simulink model "MovingAvg41"  (R2022a)
settings: Solver=FixedStepAuto  StartTime=0.0  StopTime=1500  FixedStep=1/3600  RelTol=1e-3
undefined symbols (not defined in the file or in its folder): sigbuilder_block
libraries: dspsrcs4 x1
settings Model: Creator=rupak  LastModifiedBy=rupak
settings ConfigComp: DVTestSuiteOptimization=Auto  DVDetectOutOfBounds=on  DVModelReferenceHarness=on  DVHarnessSource=Signal Editor

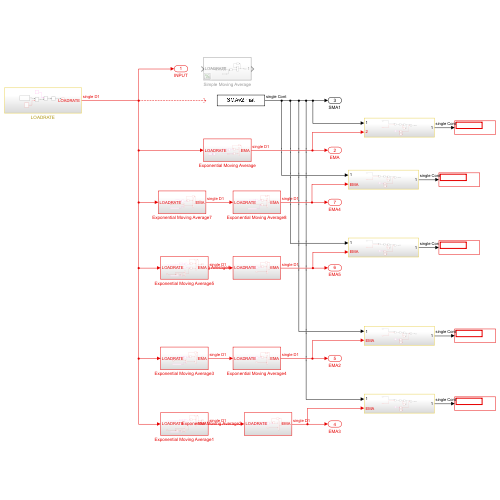
[thumbnail: Simulink's stored preview of the top-level diagram]
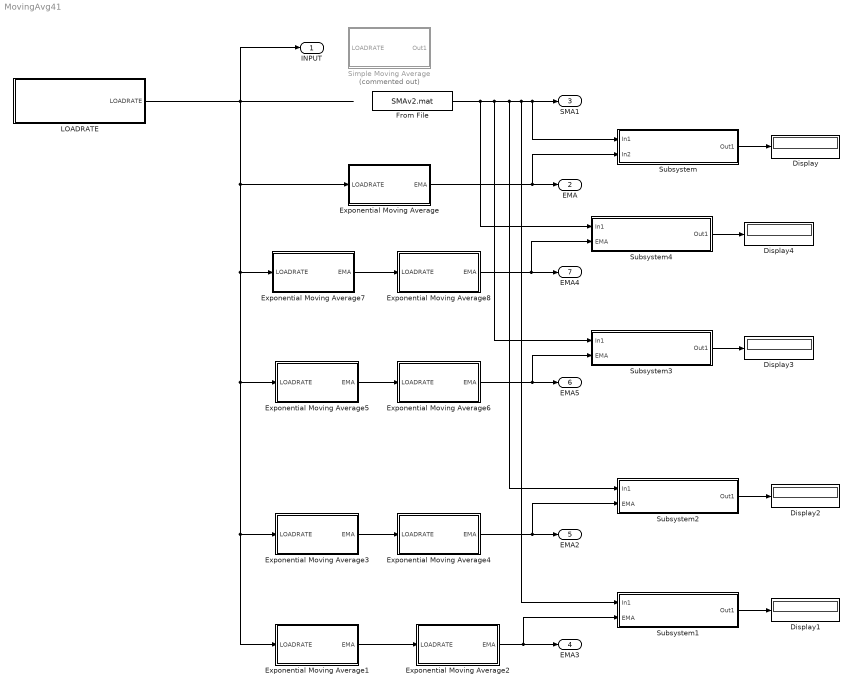
== system MovingAvg41 ==
  Display{,1..4} (5 alike) : Display
  Exponential Moving Average : Subsystem
  Exponential Moving Average1 : Subsystem
  Exponential Moving Average2 : Subsystem
  Exponential Moving Average3 : Subsystem
  Exponential Moving Average4 : Subsystem
  Exponential Moving Average5 : Subsystem
  Exponential Moving Average6 : Subsystem
  Exponential Moving Average7 : Subsystem
  Exponential Moving Average8 : Subsystem
  From File : FromFile  FileName=SMAv2.mat  SampleTime=0
  LOADRATE : Subsystem
  Simple Moving Average : Subsystem  Commented=on
  Subsystem : Subsystem
  Subsystem1 : Subsystem
  Subsystem2 : Subsystem
  Subsystem3 : Subsystem
  Subsystem4 : Subsystem
  INPUT : Outport
  EMA : Outport  Port=2
  SMA1 : Outport  Port=3
  EMA3 : Outport  Port=4
  EMA2 : Outport  Port=5
  EMA5 : Outport  Port=6
  EMA4 : Outport  Port=7
  wires:
  Exponential Moving Average/1(EMA) -> EMA/1, Subsystem/2(In2)
  Exponential Moving Average1/1(EMA) -> Exponential Moving Average2/1(LOADRATE)
  Exponential Moving Average2/1(EMA) -> EMA3/1, Subsystem1/2(EMA)
  LOADRATE/1(LOADRATE) -> INPUT/1, Exponential Moving Average3/1(LOADRATE), Exponential Moving Average1/1(LOADRATE), Exponential Moving Average5/1(LOADRATE), Exponential Moving Average7/1(LOADRATE), Exponential Moving Average/1(LOADRATE)
  Subsystem/1(Out1) -> Display/1
  Subsystem1/1(Out1) -> Display1/1
  Exponential Moving Average3/1(EMA) -> Exponential Moving Average4/1(LOADRATE)
  Exponential Moving Average4/1(EMA) -> Subsystem2/2(EMA), EMA2/1
  Subsystem2/1(Out1) -> Display2/1
  Exponential Moving Average8/1(EMA) -> Subsystem4/2(EMA), EMA4/1
  From File/1 -> Subsystem4/1(In1), Subsystem3/1(In1), Subsystem2/1(In1), Subsystem1/1(In1), Subsystem/1(In1), SMA1/1
  Subsystem4/1(Out1) -> Display4/1
  Exponential Moving Average5/1(EMA) -> Exponential Moving Average6/1(LOADRATE)
  Exponential Moving Average7/1(EMA) -> Exponential Moving Average8/1(LOADRATE)
  Exponential Moving Average6/1(EMA) -> EMA5/1, Subsystem3/2(EMA)
  Subsystem3/1(Out1) -> Display3/1

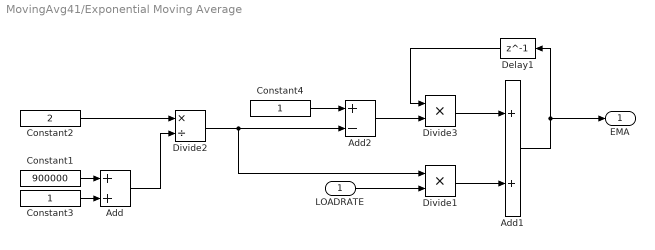
== system MovingAvg41/Exponential Moving Average ==
  LOADRATE : Inport
  Add : Sum
  Add1 : Sum
  Add2 : Sum  Inputs=+-
  Constant1 : Constant  Value=900000  OutDataTypeStr=single
  Constant2 : Constant  Value=2  OutDataTypeStr=single
  Constant3 : Constant  OutDataTypeStr=single
  Constant4 : Constant  OutDataTypeStr=single
  Delay1 : Delay  DelayLength=1  InitialCondition=60
  Divide1 : Product  Inputs=**
  Divide2 : Product  Inputs=*/
  Divide3 : Product  Inputs=**
  EMA : Outport
  wires:
  Add1/1 -> EMA/1, Delay1/1
  Divide1/1 -> Add1/2
  Constant2/1 -> Divide2/1
  Constant1/1 -> Add/1
  Constant3/1 -> Add/2
  Add/1 -> Divide2/2
  Delay1/1 -> Divide3/1
  Divide3/1 -> Add1/1
  Add2/1 -> Divide3/2
  Constant4/1 -> Add2/1
  Divide2/1 -> Add2/2, Divide1/1
  LOADRATE/1 -> Divide1/2

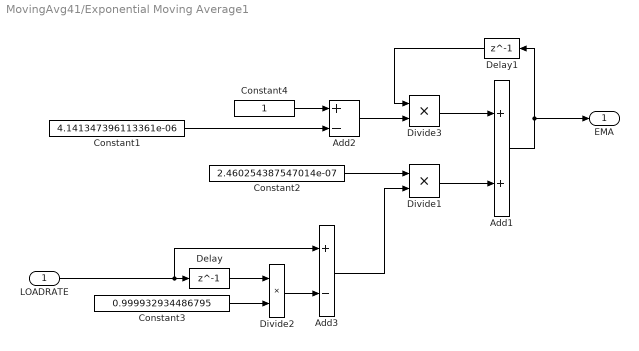
== system MovingAvg41/Exponential Moving Average1 ==
  LOADRATE : Inport
  Add1 : Sum
  Add2 : Sum  Inputs=+-
  Add3 : Sum  Inputs=+-
  Constant1 : Constant  Value=4.141347396113361e-06  OutDataTypeStr=single
  Constant2 : Constant  Value=2.460254387547014e-07  OutDataTypeStr=single
  Constant3 : Constant  Value=0.999932934486795  OutDataTypeStr=single
  Constant4 : Constant  OutDataTypeStr=single
  Delay : Delay  DelayLength=1  InitialCondition=60
  Delay1 : Delay  DelayLength=1  InitialCondition=0.000238234
  Divide1 : Product  Inputs=**
  Divide2 : Product  Inputs=**
  Divide3 : Product  Inputs=**
  EMA : Outport
  wires:
  Add1/1 -> EMA/1, Delay1/1
  Divide1/1 -> Add1/2
  Delay1/1 -> Divide3/1
  Divide3/1 -> Add1/1
  Add2/1 -> Divide3/2
  Constant4/1 -> Add2/1
  Constant1/1 -> Add2/2
  LOADRATE/1 -> Add3/1, Delay/1
  Delay/1 -> Divide2/1
  Constant3/1 -> Divide2/2
  Add3/1 -> Divide1/2
  Divide2/1 -> Add3/2
  Constant2/1 -> Divide1/1

== system MovingAvg41/Exponential Moving Average2 ==
  LOADRATE : Inport
  Add1 : Sum
  Add2 : Sum  Inputs=+-
  Constant1 : Constant  Value=3.970570935940934e-06  OutDataTypeStr=single
  Constant4 : Constant  OutDataTypeStr=single
  Delay1 : Delay  DelayLength=1  InitialCondition=60
  Divide3 : Product  Inputs=**
  EMA : Outport
  wires:
  Add1/1 -> EMA/1, Delay1/1
  LOADRATE/1 -> Add1/2
  Delay1/1 -> Divide3/1
  Divide3/1 -> Add1/1
  Add2/1 -> Divide3/2
  Constant4/1 -> Add2/1
  Constant1/1 -> Add2/2

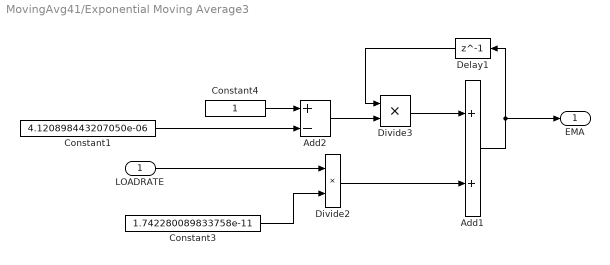
== system MovingAvg41/Exponential Moving Average3 ==
  LOADRATE : Inport
  Add1 : Sum
  Add2 : Sum  Inputs=+-
  Constant1 : Constant  Value=4.120898443207050e-06  OutDataTypeStr=single
  Constant3 : Constant  Value=1.742280089833758e-11  OutDataTypeStr=single
  Constant4 : Constant  OutDataTypeStr=single
  Delay1 : Delay  DelayLength=1  InitialCondition=0.000252816
  Divide2 : Product  Inputs=**
  Divide3 : Product  Inputs=**
  EMA : Outport
  wires:
  Add1/1 -> EMA/1, Delay1/1
  Divide2/1 -> Add1/2
  Delay1/1 -> Divide3/1
  Divide3/1 -> Add1/1
  Add2/1 -> Divide3/2
  Constant4/1 -> Add2/1
  Constant1/1 -> Add2/2
  LOADRATE/1 -> Divide2/1
  Constant3/1 -> Divide2/2

== system MovingAvg41/Exponential Moving Average4 ==
  LOADRATE : Inport
  Add1 : Sum
  Add2 : Sum  Inputs=+-
  Constant1 : Constant  Value=4.213596409140841e-06  OutDataTypeStr=single
  Constant4 : Constant  OutDataTypeStr=single
  Delay1 : Delay  DelayLength=1  InitialCondition=60
  Divide3 : Product  Inputs=**
  EMA : Outport
  wires:
  Add1/1 -> EMA/1, Delay1/1
  LOADRATE/1 -> Add1/2
  Delay1/1 -> Divide3/1
  Divide3/1 -> Add1/1
  Add2/1 -> Divide3/2
  Constant4/1 -> Add2/1
  Constant1/1 -> Add2/2

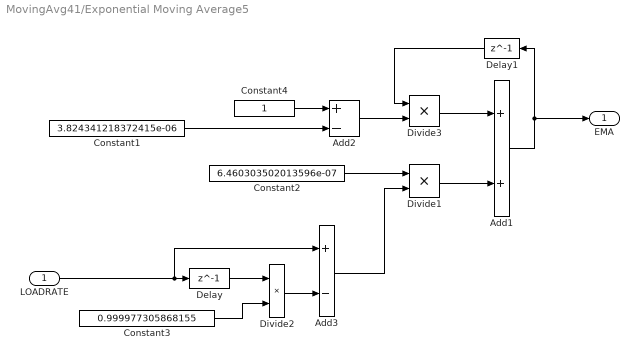
== system MovingAvg41/Exponential Moving Average5 ==
  LOADRATE : Inport
  Add1 : Sum
  Add2 : Sum  Inputs=+-
  Add3 : Sum  Inputs=+-
  Constant1 : Constant  Value=3.824341218372415e-06  OutDataTypeStr=single
  Constant2 : Constant  Value=6.460303502013596e-07  OutDataTypeStr=single
  Constant3 : Constant  Value=0.999977305868155  OutDataTypeStr=single
  Constant4 : Constant  OutDataTypeStr=single
  Delay : Delay  DelayLength=1  InitialCondition=60
  Delay1 : Delay  DelayLength=1  InitialCondition=0.000229104
  Divide1 : Product  Inputs=**
  Divide2 : Product  Inputs=**
  Divide3 : Product  Inputs=**
  EMA : Outport
  wires:
  Add1/1 -> EMA/1, Delay1/1
  Divide1/1 -> Add1/2
  Delay1/1 -> Divide3/1
  Divide3/1 -> Add1/1
  Add2/1 -> Divide3/2
  Constant4/1 -> Add2/1
  Constant1/1 -> Add2/2
  LOADRATE/1 -> Add3/1, Delay/1
  Delay/1 -> Divide2/1
  Constant3/1 -> Divide2/2
  Add3/1 -> Divide1/2
  Divide2/1 -> Add3/2
  Constant2/1 -> Divide1/1

== system MovingAvg41/Exponential Moving Average6 ==
  LOADRATE : Inport
  Add1 : Sum
  Add2 : Sum  Inputs=+-
  Constant1 : Constant  Value=3.818393625660592e-06  OutDataTypeStr=single
  Constant4 : Constant  OutDataTypeStr=single
  Delay1 : Delay  DelayLength=1  InitialCondition=60
  Divide3 : Product  Inputs=**
  EMA : Outport
  wires:
  Add1/1 -> EMA/1, Delay1/1
  LOADRATE/1 -> Add1/2
  Delay1/1 -> Divide3/1
  Divide3/1 -> Add1/1
  Add2/1 -> Divide3/2
  Constant4/1 -> Add2/1
  Constant1/1 -> Add2/2

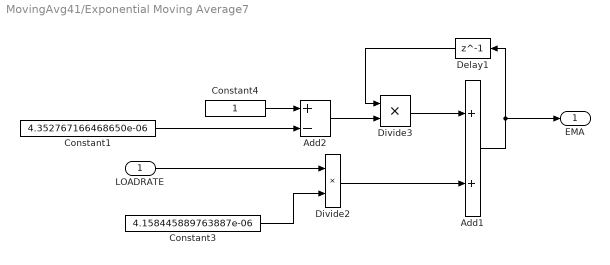
== system MovingAvg41/Exponential Moving Average7 ==
  LOADRATE : Inport
  Add1 : Sum
  Add2 : Sum  Inputs=+-
  Constant1 : Constant  Value=4.352767166468650e-06  OutDataTypeStr=single
  Constant3 : Constant  Value=4.158445889763887e-06  OutDataTypeStr=single
  Constant4 : Constant  OutDataTypeStr=single
  Delay1 : Delay  DelayLength=1  InitialCondition=56.8729
  Divide2 : Product  Inputs=**
  Divide3 : Product  Inputs=**
  EMA : Outport
  wires:
  Add1/1 -> EMA/1, Delay1/1
  Divide2/1 -> Add1/2
  Delay1/1 -> Divide3/1
  Divide3/1 -> Add1/1
  Add2/1 -> Divide3/2
  Constant4/1 -> Add2/1
  Constant1/1 -> Add2/2
  LOADRATE/1 -> Divide2/1
  Constant3/1 -> Divide2/2

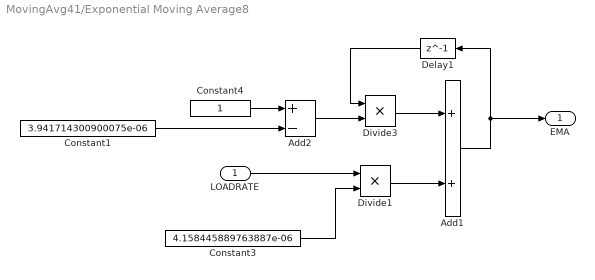
== system MovingAvg41/Exponential Moving Average8 ==
  LOADRATE : Inport
  Add1 : Sum
  Add2 : Sum  Inputs=+-
  Constant1 : Constant  Value=3.941714300900075e-06  OutDataTypeStr=single
  Constant3 : Constant  Value=4.158445889763887e-06  OutDataTypeStr=single
  Constant4 : Constant  OutDataTypeStr=single
  Delay1 : Delay  DelayLength=1  InitialCondition=60
  Divide1 : Product  Inputs=**
  Divide3 : Product  Inputs=**
  EMA : Outport
  wires:
  Add1/1 -> EMA/1, Delay1/1
  Delay1/1 -> Divide3/1
  Divide3/1 -> Add1/1
  Add2/1 -> Divide3/2
  Constant4/1 -> Add2/1
  Constant1/1 -> Add2/2
  Constant3/1 -> Divide1/2
  LOADRATE/1 -> Divide1/1
  Divide1/1 -> Add1/2

== system MovingAvg41/LOADRATE ==
  Add : Sum
  Constant : Constant  OutDataTypeStr=single
  Divide : Product  Inputs=**  OutDataTypeStr=Inherit: Same as first input
  Random Source : dspsrcs4/Random Source  SrcType=Uniform  NormMethod=Sum of uniform values  CltLength=12  MinVal=-100  MaxVal=100  MeanVal=0  VarVal=1  RepMode=Not repeatable  rawSeed=1  IsInherit=off  SampMode=Discrete  SampTime=1/3600  SampFrame=1  DataType=Single  OutComplex=Real  OutputFrames=off
  Saturation : Saturate  UpperLimit=100  LowerLimit=0
  Signal Builder1 : Subsystem  Tag=STV Subsys  LoadFcn=sigbuilder_block('load');  StartFcn=sigbuilder_block('start');  StopFcn=sigbuilder_block('stop');  ClipboardFcn=sigbuilder_block('clipboard');  mask(Sigbuilder block){tuvar=[0:10]}
      mask help: Simulink:masks:SigbuilderBlock_MD
      mask init:
      | if ~strcmp(get_param(bdroot(gcbh),'SimulationStatus'),'stopped') tuvar = sigbuilder_block('maskInit'); end
      settings: CopyFcn=sigbuilder_block('copy');  DeleteFcn=sigbuilder_block('delete');  ModelCloseFcn=sigbuilder_block('modelClose');  PreSaveFcn=sigbuilder_block('preSave');  PauseFcn=sigbuilder_block('pause');  ContinueFcn=sigbuilder_block('continue');  NameChangeFcn=sigbuilder_block('namechange');  OpenFcn=sigbuilder_block('open',[6 -8.25 1428 635.25 ]);  CloseFcn=sigbuilder_block('close');
      mask Display: plot(0, 0, 100, 100,[2, 2, 32, 32, 2], [68, 8, 8, 68, 68],[32, 2], [38, 38], [32, 19, 2],[53, 60, 44], [32, 17, 17, 2],[16, 16, 31, 31]);txt = getActiveGroup(gcbh);text(2, 100, txt,'verticalAlignment', 'top');
  LOADRATE : Outport  SampleTime=1/3600
  wires:
  Random Source/1 -> Add/2
  Signal Builder1/1(Signal 1) -> Add/1
  Add/1 -> Divide/2
  Constant/1 -> Divide/1
  Saturation/1 -> LOADRATE/1
  Divide/1 -> Saturation/1

== system MovingAvg41/Simple Moving Average ==
  LOADRATE : Inport
  Add : Sum  Inputs=+-
  Add1 : Sum
  Constant : Constant  Value=900000  OutDataTypeStr=single
  Delay : Delay  DelayLength=900000  InitialCondition=60
  Delay1 : Delay  DelayLength=1  InitialCondition=60
  Divide : Product  Inputs=*/
  Out1 : Outport
  wires:
  Delay/1 -> Add/2
  Delay1/1 -> Add1/1
  Constant/1 -> Divide/2
  LOADRATE/1 -> Delay/1, Add/1
  Add/1 -> Divide/1
  Add1/1 -> Out1/1, Delay1/1
  Divide/1 -> Add1/2

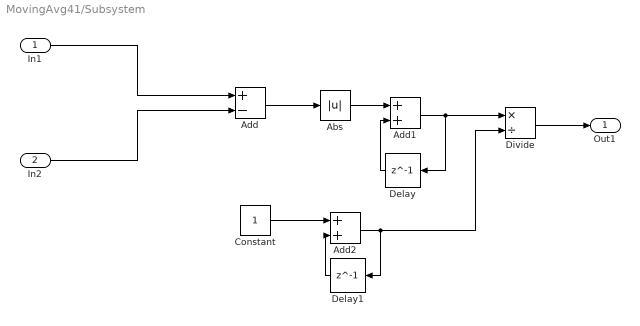
== system MovingAvg41/Subsystem ==
  In1 : Inport
  In2 : Inport  Port=2
  Abs : Abs  SaturateOnIntegerOverflow=off
  Add : Sum  Inputs=+-
  Add1 : Sum
  Add2 : Sum
  Constant : Constant  OutDataTypeStr=single
  Delay : Delay  DelayLength=1
  Delay1 : Delay  DelayLength=1
  Divide : Product  Inputs=*/
  Out1 : Outport
  wires:
  Add/1 -> Abs/1
  Add2/1 -> Divide/2, Delay1/1
  Delay1/1 -> Add2/2
  In1/1 -> Add/1
  Add1/1 -> Delay/1, Divide/1
  Delay/1 -> Add1/2
  In2/1 -> Add/2
  Abs/1 -> Add1/1
  Constant/1 -> Add2/1
  Divide/1 -> Out1/1

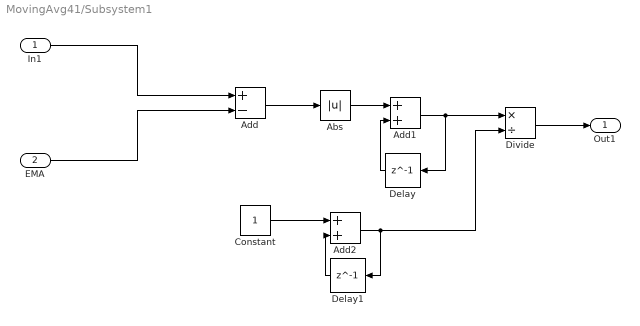
== system MovingAvg41/Subsystem1 ==
  In1 : Inport
  EMA : Inport  Port=2
  Abs : Abs  SaturateOnIntegerOverflow=off
  Add : Sum  Inputs=+-
  Add1 : Sum
  Add2 : Sum
  Constant : Constant  OutDataTypeStr=single
  Delay : Delay  DelayLength=1
  Delay1 : Delay  DelayLength=1
  Divide : Product  Inputs=*/
  Out1 : Outport
  wires:
  Divide/1 -> Out1/1
  Constant/1 -> Add2/1
  Abs/1 -> Add1/1
  EMA/1 -> Add/2
  Delay/1 -> Add1/2
  Add1/1 -> Divide/1, Delay/1
  In1/1 -> Add/1
  Delay1/1 -> Add2/2
  Add2/1 -> Delay1/1, Divide/2
  Add/1 -> Abs/1

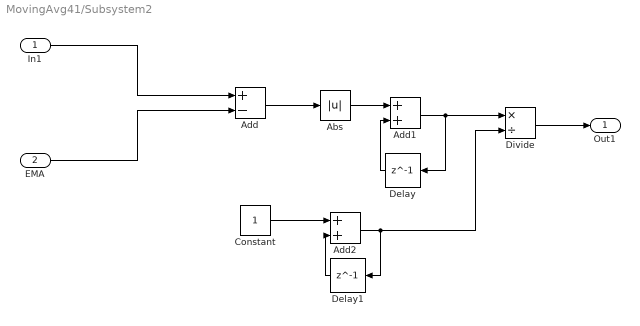
== system MovingAvg41/Subsystem2 ==
  In1 : Inport
  EMA : Inport  Port=2
  Abs : Abs  SaturateOnIntegerOverflow=off
  Add : Sum  Inputs=+-
  Add1 : Sum
  Add2 : Sum
  Constant : Constant  OutDataTypeStr=single
  Delay : Delay  DelayLength=1
  Delay1 : Delay  DelayLength=1
  Divide : Product  Inputs=*/
  Out1 : Outport
  wires:
  Divide/1 -> Out1/1
  Constant/1 -> Add2/1
  Abs/1 -> Add1/1
  EMA/1 -> Add/2
  Delay/1 -> Add1/2
  Add1/1 -> Divide/1, Delay/1
  In1/1 -> Add/1
  Delay1/1 -> Add2/2
  Add2/1 -> Delay1/1, Divide/2
  Add/1 -> Abs/1

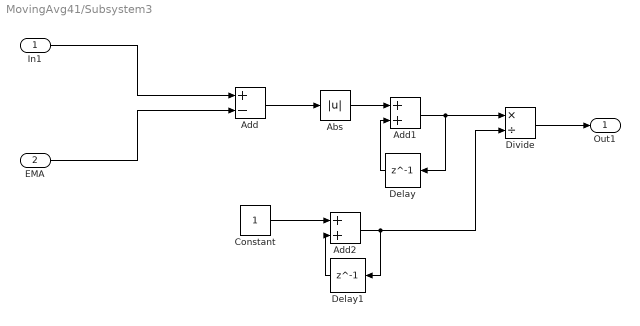
== system MovingAvg41/Subsystem3 ==
  In1 : Inport
  EMA : Inport  Port=2
  Abs : Abs  SaturateOnIntegerOverflow=off
  Add : Sum  Inputs=+-
  Add1 : Sum
  Add2 : Sum
  Constant : Constant  OutDataTypeStr=single
  Delay : Delay  DelayLength=1
  Delay1 : Delay  DelayLength=1
  Divide : Product  Inputs=*/
  Out1 : Outport
  wires:
  Divide/1 -> Out1/1
  Constant/1 -> Add2/1
  Abs/1 -> Add1/1
  EMA/1 -> Add/2
  Delay/1 -> Add1/2
  Add1/1 -> Divide/1, Delay/1
  In1/1 -> Add/1
  Delay1/1 -> Add2/2
  Add2/1 -> Delay1/1, Divide/2
  Add/1 -> Abs/1

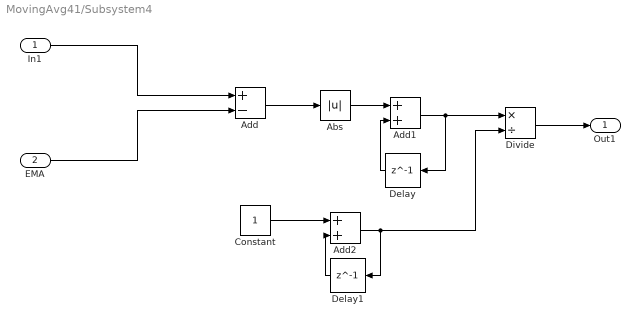
== system MovingAvg41/Subsystem4 ==
  In1 : Inport
  EMA : Inport  Port=2
  Abs : Abs  SaturateOnIntegerOverflow=off
  Add : Sum  Inputs=+-
  Add1 : Sum
  Add2 : Sum
  Constant : Constant  OutDataTypeStr=single
  Delay : Delay  DelayLength=1
  Delay1 : Delay  DelayLength=1
  Divide : Product  Inputs=*/
  Out1 : Outport
  wires:
  Divide/1 -> Out1/1
  Constant/1 -> Add2/1
  Abs/1 -> Add1/1
  EMA/1 -> Add/2
  Delay/1 -> Add1/2
  Add1/1 -> Divide/1, Delay/1
  In1/1 -> Add/1
  Delay1/1 -> Add2/2
  Add2/1 -> Delay1/1, Divide/2
  Add/1 -> Abs/1

== system MovingAvg41/LOADRATE/Signal Builder1 ==
  Demux : Demux  Tag=STV Demux  Outputs=1
      settings: DisplayOption=none
  FromWs : FromWorkspace  Tag=STV FromWs  VariableName=tuvar
      SigBuilderData=|
      | common.afterFinalStr = 'Extrapolate'
      | common.sampleTime = 0
      | dataSet.timeRange = [0 1500]
      | dataSet.name = 'Group 1'
      | sbobj.Groups.Name = 'Group 1'
      | sbobj.Groups.Signals.Name = 'Signal 1'
      | sbobj.Groups.Signals.XData = [0 4 4 10 12 16 18 20 24 30 36 40 44 50 56 60 60 64 64 70 74 78 80 82 86 88 88 90 92 98 104 108 112 118 122 122 128 128 132 138 144 150 154 158 160 162 166 170 174 176 180 182 184 190 196 200 202 202 208 208 216 226 232 240 240 250 250 260 266 278 278 284 292 296 300 304 310 316 322 326 338 346 356 362 362 368 368 374 374 378 384 392 400 400 406 406 414 414 420 424 430 432 438 442 446 450 458 464 470 476 482 487 489 490 496 500 508 518 528 536 546 552 558 562 570 582 588 592 598 606 620 626 634 644 650 664 673 674 682 696 706 706 717 717 724 734 744 756 756 764 772 780 790 800 808 816 826 834 834 844 856 864 864 872 880 890 904 972 994 997 1006 1006 1016 1016 1024 1025 1026 1034 1059 1072 1092 1116 1126 1134 1142 1156 1160 1166 1176 1182 1190 1198 1208 1220 1228 1235 1246 1258 1265 1277 1287 1297 1308 1323 1332 1342 1347 1355 1361 1371 1379 1389 1402 1408 1415 1422 1435 1439 1446 1453 1469 1475 1485 1485 1492 1492 1495 1495 1500]
      | sbobj.Groups.Signals.YData = [20.4 96.2 94.4 96.2 91.6 91.6 90 90.2 87.8 89.2 91 87.8 90.2 87 84 81 79.6 77 77.6 71.6 70 68.2 66.2 66 65.6 64 65.2 65 63.4 64.8 63.6 63.2 64.2 62.4 62.6 62 60.4 61 60.8 60 59.8 59.4 60.6 58.8 59.2 59.4 60.4 60.6 61.2 58.6 61.4 59.4 60.4 59.4 60.6 62.4 59.8 59.6 60.4 59 60.6 58.8 59.6 58.6 58.4 58.6 57.8 58.2 58.2 59.2 60 59.2 59.4 59 58.4 58.2 59.4 57.8 59.2 59.4 60.2 59 59.8 58.4 59.8 56.6 59.2 58.4 58.6 56.6 60.6 60.8 61.8 61 62.4 61.2 61.2 61.8 61.2 63.4 63.2 63.2 62.4 63.4 64 64.8 65.2 64.4 65.8 68.2 69.8 72.4 74 77.8 80.4 82.8 82.6 82.6 83.2 83.4 83.2 82.2 83 80 80.6 73.2 69 69.2 67 67 67 66.6 66.6 66.4 66.2 66.4 66 66 66.6 66.2 69.2 70.6 67.8 68 69.2 67.2 67 68.4 68.2 70.8 70.6 70.2 70.2 70.4 69.4 69.4 69.4 71.2 70.8 70.6 71 70.8 71 71.2 71.6 70.8 71 71.2 69.2 69.2 69.8 68.8 70.8 71.8 69.6 71.8 70.4 69.8 70.6 69.2 69.4 68.8 69.4 65.2 66.6 71.4 71.8 74.2 74.2 73 76.8 77.6 77.8 77.6 76.2 74.6 76 75.2 75.6 73.8 75.8 76.4 76.2 77 72.8 70.6 70.6 66 67.8 64.2 65.2 65.2 64.8 63.6 63.2 63 63.2 65 63.8 64.2 65 64.6 65.2 65.8 68 65.6 63.8 66.6 67.2]
      | sbobj.Groups.TimeRange = [0 1500]
  Signal 1 : Outport  Tag=STV Outport
  wires:
  Demux/1 -> Signal 1/1
  FromWs/1 -> Demux/1
